simulink model "Vasca_1es"  (R2022a)
settings: Solver=VariableStepAuto  StartTime=0.0  StopTime=3000  RelTol=1e-3
values from neighbouring files (symbols this model uses):
  Area = 0.08    [vettori_vasca.m]
  Au = 43*1e-6    (= 4.3e-05)    [vettori_vasca.m]
  g = 9.8    [vettori_vasca.m]
  hu = -0.095    [vettori_vasca.m]
  L_T = 0:0.01:0.2    [vettori_vasca.m]
  Q_A = 1e-6*[0 8.8 24.6 42.0 57.1 72.4 86.1 102.3 117.6 132.0 144.9]    [vettori_vasca.m]
  Tn_A = 0:0.5:5    [vettori_vasca.m]
  Tn_T = [4.5221 4.4452 4.2412 3.9653 3.7932 3.5179 3.2742 3.0624 2.8349 2.5936 2.3522 2.1423 1.9151 1.6591 1.4251 1.1892 0.9053 0.7329 0.4750 0.2664 0.0471]    [vettori_vasca.m]
  x0 = 0    [vettori_vasca.m]
settings Model: Creator=cl481357  LastModifiedBy=cl481357

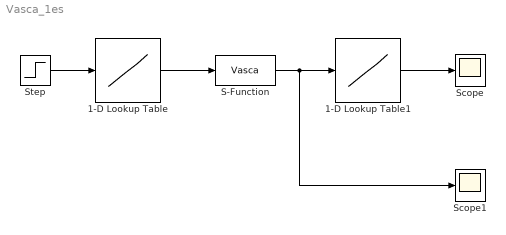
== system Vasca_1es ==
  1-D Lookup Table : Lookup_n-D  NumberOfTableDimensions=1  BreakpointsForDimension1=Tn_A  Table=Q_A  InternalRulePriority=Speed  RndMeth=Simplest
  1-D Lookup Table1 : Lookup_n-D  NumberOfTableDimensions=1  BreakpointsForDimension1=L_T  Table=Tn_T  InternalRulePriority=Speed  RndMeth=Simplest
  S-Function : S-Function  FunctionName=Vasca  Parameters=x0,Area,Au,g,hu  SFunctionDeploymentMode=off  EnableBusSupport=off
  Scope : Scope
  Scope1 : Scope
  Step : Step  After=3.2  SampleTime=0
  wires:
  1-D Lookup Table/1 -> S-Function/1
  S-Function/1 -> Scope1/1, 1-D Lookup Table1/1
  Step/1 -> 1-D Lookup Table/1
  1-D Lookup Table1/1 -> Scope/1
